simulink model "pmsm_sensorless_control"  (R2021a)
settings: Solver=VariableStepAuto  StartTime=0.0  StopTime=10.0  RelTol=1e-3
undefined symbols (not defined in the file): induction_motor, sin_cos_calculator
libraries: eeTransforms x2
settings Model: Creator=danesh  LastModifiedBy=danesh

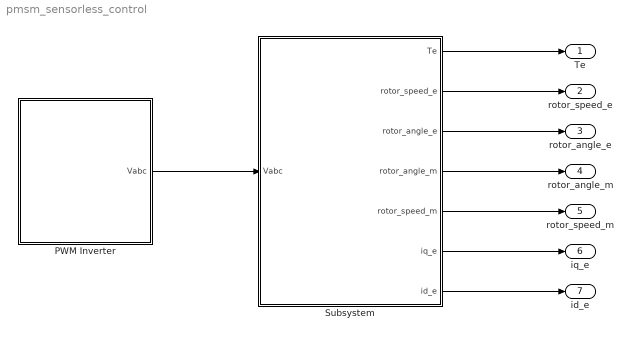
== system pmsm_sensorless_control ==
  PWM Inverter : Subsystem
  Subsystem : Subsystem
  Te : Outport  VectorParamsAs1DForOutWhenUnconnected=off
  rotor_speed_e : Outport  Port=2  VectorParamsAs1DForOutWhenUnconnected=off
  rotor_angle_e : Outport  Port=3  VectorParamsAs1DForOutWhenUnconnected=off
  rotor_angle_m : Outport  Port=4  VectorParamsAs1DForOutWhenUnconnected=off
  rotor_speed_m : Outport  Port=5  VectorParamsAs1DForOutWhenUnconnected=off
  iq_e : Outport  Port=6  VectorParamsAs1DForOutWhenUnconnected=off
  "id_e " : Outport  Port=7  VectorParamsAs1DForOutWhenUnconnected=off
  wires:
  Subsystem/6(iq_e) -> iq_e/1
  Subsystem/3(rotor_angle_e) -> rotor_angle_e/1
  Subsystem/5(rotor_speed_m) -> rotor_speed_m/1
  Subsystem/4(rotor_angle_m) -> rotor_angle_m/1
  Subsystem/2(rotor_speed_e) -> rotor_speed_e/1
  Subsystem/1(Te) -> Te/1
  PWM Inverter/1(Vabc) -> Subsystem/1(Vabc)
  Subsystem/7("id_e ") -> "id_e "/1

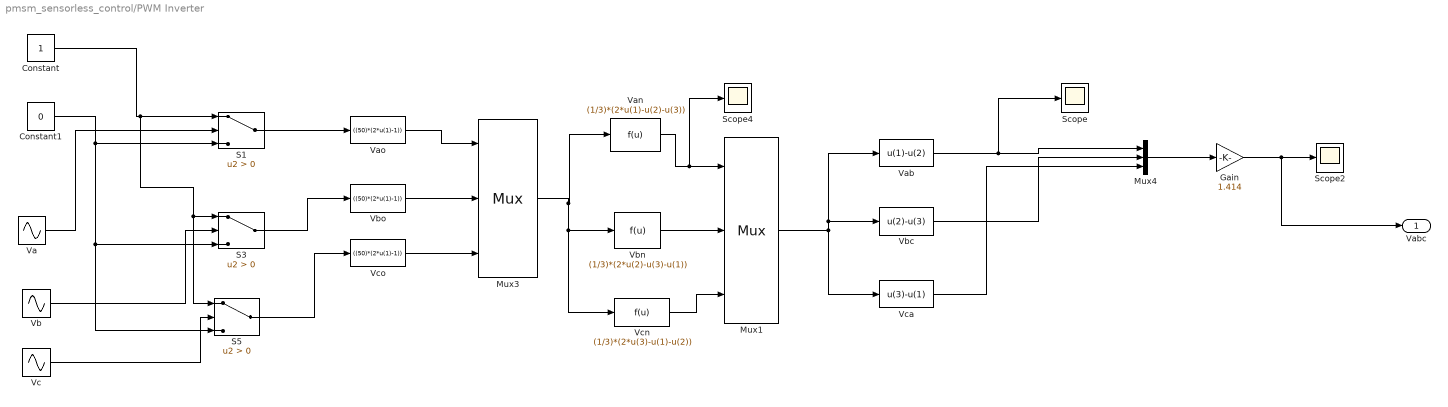
== system pmsm_sensorless_control/PWM Inverter ==
  Constant : Constant
  Constant1 : Constant  Value=0
  Gain : Gain  Gain=1.414
  Mux1 : Mux  Inputs=3
  Mux3 : Mux  Inputs=3
  Mux4 : Mux  Inputs=3
  S1 : Switch  Criteria=u2 > Threshold
  S3 : Switch  Criteria=u2 > Threshold
  S5 : Switch  Criteria=u2 > Threshold
  Scope : Scope
  Scope2 : Scope
  Scope4 : Scope
  Va : Sin  Frequency=2*pi*50  SampleTime=0
  Vab : Fcn  Expr=u(1)-u(2)
  Van : Fcn  Expr=(1/3)*(2*u(1)-u(2)-u(3))
  Vao : Fcn  Expr=((50)*(2*u(1)-1))
  Vb : Sin  Frequency=2*pi*50  Phase=-2.0904  SampleTime=0
  Vbc : Fcn  Expr=u(2)-u(3)
  Vbn : Fcn  Expr=(1/3)*(2*u(2)-u(3)-u(1))
  Vbo : Fcn  Expr=((50)*(2*u(1)-1))
  Vc : Sin  Frequency=2*pi*50  Phase=-4.188  SampleTime=0
  Vca : Fcn  Expr=u(3)-u(1)
  Vcn : Fcn  Expr=(1/3)*(2*u(3)-u(1)-u(2))
  Vco : Fcn  Expr=((50)*(2*u(1)-1))
  Vabc : Outport  VectorParamsAs1DForOutWhenUnconnected=off
  wires:
  S5/1 -> Vco/1
  S1/1 -> Vao/1
  Vca/1 -> Mux4/3
  Vc/1 -> S5/2
  Vb/1 -> S3/2
  Vab/1 -> Scope/1, Mux4/1
  Vbo/1 -> Mux3/2
  Van/1 -> Scope4/1, Mux1/1
  Mux4/1 -> Gain/1
  Gain/1 -> Vabc/1, Scope2/1
  Constant/1 -> S3/1, S5/1, S1/1
  Vco/1 -> Mux3/3
  Constant1/1 -> S1/3, S3/3, S5/3
  Mux3/1 -> Van/1, Vcn/1, Vbn/1
  S3/1 -> Vbo/1
  Mux1/1 -> Vbc/1, Vab/1, Vca/1
  Vao/1 -> Mux3/1
  Va/1 -> S1/2
  Vbn/1 -> Mux1/2
  Vcn/1 -> Mux1/3
  Vbc/1 -> Mux4/2

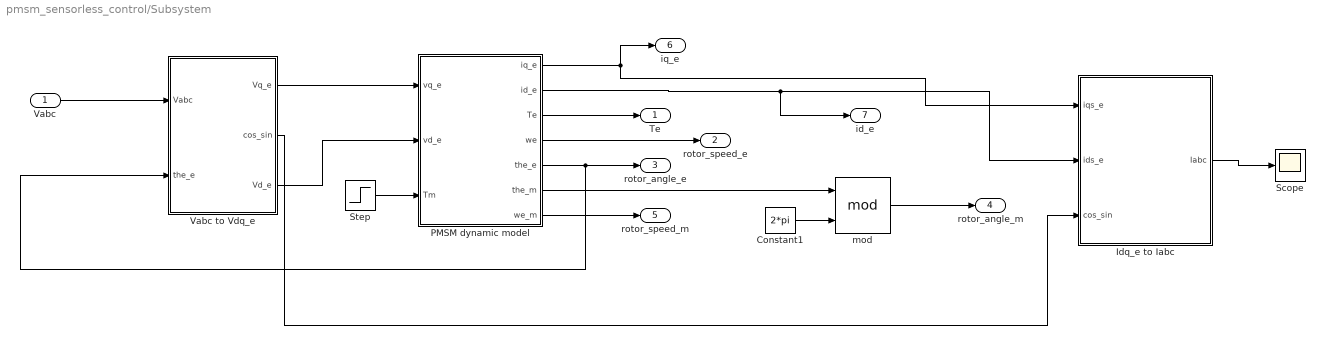
== system pmsm_sensorless_control/Subsystem ==
  Vabc : Inport
  Constant1 : Constant  Value=2*pi
  Idq_e to Iabc : Subsystem
  PMSM dynamic model : Subsystem
  Scope : Scope
  Step : Step  Time=3  SampleTime=0
  Vabc to Vdq_e : Subsystem
  mod : Math  Operator=mod  SignedPower=on  SaturateOnIntegerOverflow=on
  Te : Outport  VectorParamsAs1DForOutWhenUnconnected=off
  rotor_speed_e : Outport  Port=2  VectorParamsAs1DForOutWhenUnconnected=off
  rotor_angle_e : Outport  Port=3  VectorParamsAs1DForOutWhenUnconnected=off
  rotor_angle_m : Outport  Port=4  VectorParamsAs1DForOutWhenUnconnected=off
  rotor_speed_m : Outport  Port=5  VectorParamsAs1DForOutWhenUnconnected=off
  iq_e : Outport  Port=6  VectorParamsAs1DForOutWhenUnconnected=off
  "id_e " : Outport  Port=7  VectorParamsAs1DForOutWhenUnconnected=off
  wires:
  PMSM dynamic model/4(we) -> rotor_speed_e/1
  Idq_e to Iabc/1(Iabc) -> Scope/1
  PMSM dynamic model/2(id_e) -> "id_e "/1, Idq_e to Iabc/2(ids_e)
  mod/1 -> rotor_angle_m/1
  PMSM dynamic model/7(we_m) -> rotor_speed_m/1
  PMSM dynamic model/5(the_e) -> rotor_angle_e/1, Vabc to Vdq_e/2(the_e)
  PMSM dynamic model/6(the_m) -> mod/1
  Step/1 -> PMSM dynamic model/3(Tm)
  PMSM dynamic model/1(iq_e) -> iq_e/1, Idq_e to Iabc/1(iqs_e)
  PMSM dynamic model/3(Te) -> Te/1
  Constant1/1 -> mod/2
  Vabc to Vdq_e/1(Vq_e) -> PMSM dynamic model/1(vq_e)
  Vabc to Vdq_e/2(cos_sin) -> Idq_e to Iabc/3(cos_sin)
  Vabc to Vdq_e/3(Vd_e) -> PMSM dynamic model/2(vd_e)
  Vabc/1 -> Vabc to Vdq_e/1(Vabc)

== system pmsm_sensorless_control/Subsystem/Idq_e to Iabc ==
  iqs_e : Inport
  ids_e : Inport  Port=2
  cos_sin : Inport  Port=3
  Constant2 : Constant  Value=0
  Demux : Demux  Outputs=2
  Subsystem : Subsystem
  de-qe to ds-qs : Subsystem  AncestorBlock=induction_motor/de-qe to ds-qs
  Iabc : Outport  VectorParamsAs1DForOutWhenUnconnected=off
  wires:
  de-qe to ds-qs/1(qs_s) -> Subsystem/1(q_s)
  de-qe to ds-qs/2(ds_s) -> Subsystem/2(d_s)
  Constant2/1 -> Subsystem/4(thetha_degree)
  Subsystem/1(abc) -> Iabc/1
  iqs_e/1 -> de-qe to ds-qs/1(qs_e)
  ids_e/1 -> de-qe to ds-qs/2(ds_e)
  Demux/1 -> de-qe to ds-qs/3(cos Oe)
  Demux/2 -> de-qe to ds-qs/4(Sin Oe)
  cos_sin/1 -> Demux/1

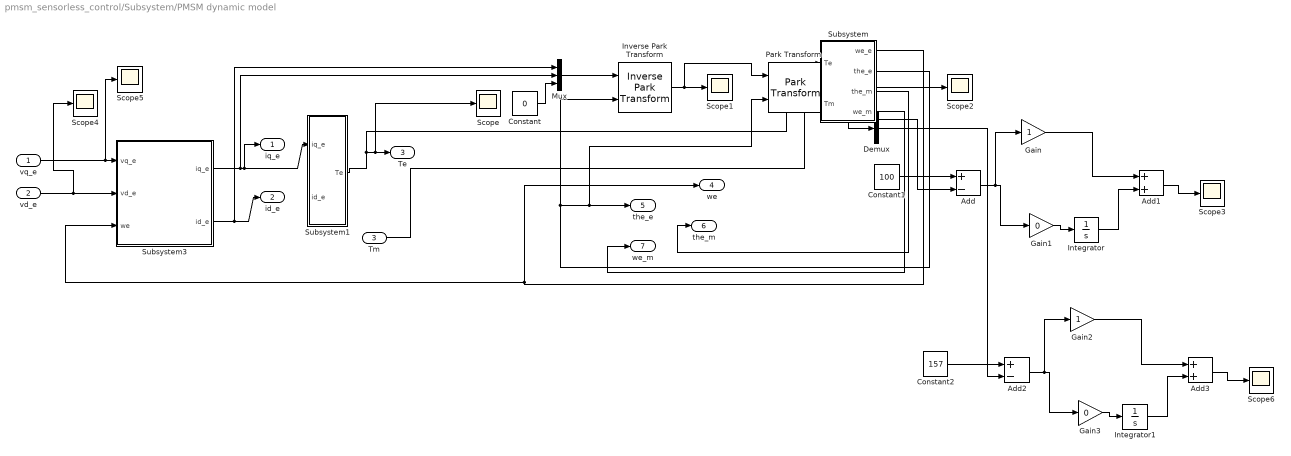
== system pmsm_sensorless_control/Subsystem/PMSM dynamic model ==
  vq_e : Inport
  vd_e : Inport  Port=2
  Tm : Inport  Port=3
  Add : Sum  Inputs=+-
  Add1 : Sum
  Add2 : Sum  Inputs=+-
  Add3 : Sum
  Constant : Constant  Value=0
  Constant1 : Constant  Value=100
  Constant2 : Constant  Value=157
  Demux : Demux  Outputs=3
  Gain : Gain
  Gain1 : Gain  Gain=0
  Gain2 : Gain
  Gain3 : Gain  Gain=0
  Integrator : Integrator
  Integrator1 : Integrator
  Inverse Park Transform : eeTransforms/Inverse Park Transform  AxisAlignment=Q-axis  PowerInvariant=off
  Mux : Mux  Inputs=3
  Park Transform : eeTransforms/Park Transform  AxisAlignment=Q-axis  PowerInvariant=off
  Scope{,1..6} (7 alike) : Scope
  Subsystem : Subsystem
  Subsystem1 : Subsystem
  Subsystem3 : Subsystem
  iq_e : Outport  VectorParamsAs1DForOutWhenUnconnected=off
  id_e : Outport  Port=2  VectorParamsAs1DForOutWhenUnconnected=off
  Te : Outport  Port=3  VectorParamsAs1DForOutWhenUnconnected=off
  we : Outport  Port=4  VectorParamsAs1DForOutWhenUnconnected=off
  the_e : Outport  Port=5  VectorParamsAs1DForOutWhenUnconnected=off
  the_m : Outport  Port=6  VectorParamsAs1DForOutWhenUnconnected=off
  we_m : Outport  Port=7  VectorParamsAs1DForOutWhenUnconnected=off
  wires:
  Subsystem1/1(Te) -> Subsystem/1(Te), Scope/1, Te/1
  Subsystem3/1(iq_e) -> Mux/2, Subsystem1/1(iq_e), iq_e/1
  Subsystem3/2(id_e) -> Mux/1, id_e/1
  Tm/1 -> Subsystem/2(Tm)
  vq_e/1 -> Scope5/1, Subsystem3/1(vq_e)
  vd_e/1 -> Scope4/1, Subsystem3/2(vd_e)
  Subsystem/2(the_e) -> Inverse Park Transform/2, Park Transform/2, the_e/1
  Subsystem/1(we_e) -> we/1, Subsystem3/3(we)
  Subsystem/3(the_m) -> the_m/1
  Subsystem/4(we_m) -> we_m/1
  Mux/1 -> Inverse Park Transform/1
  Constant/1 -> Mux/3
  Inverse Park Transform/1 -> Park Transform/1, Scope1/1
  Park Transform/1 -> Demux/1, Scope2/1
  Demux/1 -> Add/2
  Constant1/1 -> Add/1
  Add/1 -> Gain/1, Gain1/1
  Gain1/1 -> Integrator/1
  Gain/1 -> Add1/1
  Integrator/1 -> Add1/2
  Add1/1 -> Scope3/1
  Gain2/1 -> Add3/1
  Add3/1 -> Scope6/1
  Gain3/1 -> Integrator1/1
  Demux/2 -> Add2/2
  Constant2/1 -> Add2/1
  Add2/1 -> Gain2/1, Gain3/1
  Integrator1/1 -> Add3/2

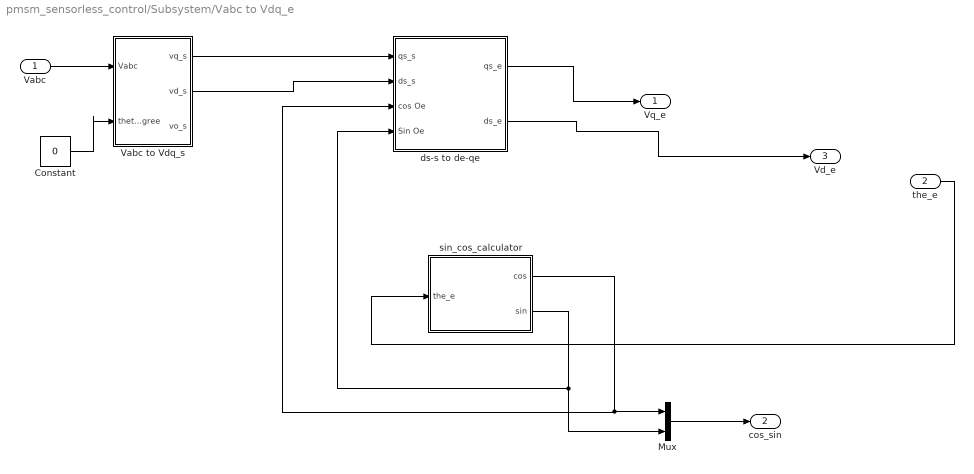
== system pmsm_sensorless_control/Subsystem/Vabc to Vdq_e ==
  Vabc : Inport
  the_e : Inport  Port=2
  Constant : Constant  Value=0
  Mux : Mux  Inputs=2
  Vabc to Vdq_s : Subsystem
  ds-s to de-qe : Subsystem  AncestorBlock=induction_motor/ds-s to de-qe
  sin_cos_calculator : Subsystem  AncestorBlock=induction_motor/sin_cos_calculator
  Vq_e : Outport  VectorParamsAs1DForOutWhenUnconnected=off
  cos_sin : Outport  Port=2  VectorParamsAs1DForOutWhenUnconnected=off
  Vd_e : Outport  Port=3  VectorParamsAs1DForOutWhenUnconnected=off
  wires:
  Mux/1 -> cos_sin/1
  sin_cos_calculator/1(cos) -> ds-s to de-qe/3(cos Oe), Mux/1
  Constant/1 -> Vabc to Vdq_s/2(thetha_degree)
  sin_cos_calculator/2(sin) -> Mux/2, ds-s to de-qe/4(Sin Oe)
  Vabc to Vdq_s/2(vd_s) -> ds-s to de-qe/2(ds_s)
  Vabc to Vdq_s/1(vq_s) -> ds-s to de-qe/1(qs_s)
  Vabc/1 -> Vabc to Vdq_s/1(Vabc)
  ds-s to de-qe/1(qs_e) -> Vq_e/1
  ds-s to de-qe/2(ds_e) -> Vd_e/1
  the_e/1 -> sin_cos_calculator/1(the_e)

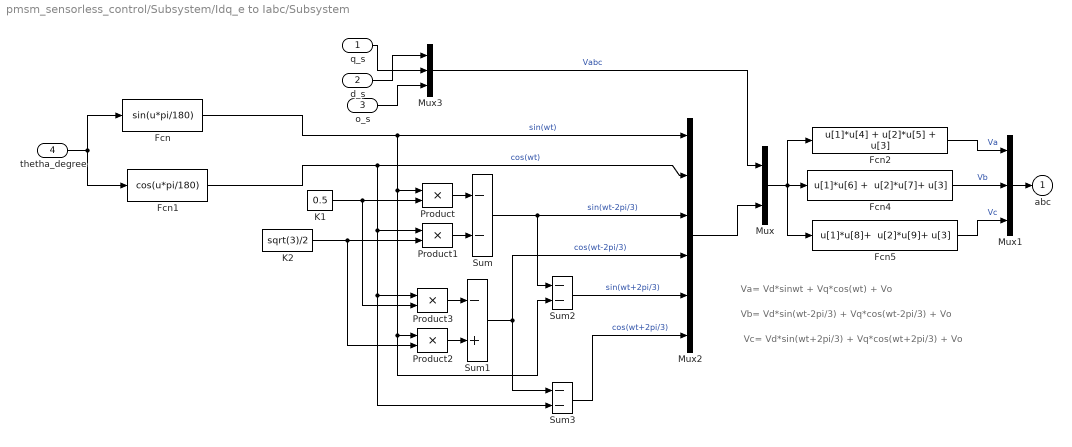
== system pmsm_sensorless_control/Subsystem/Idq_e to Iabc/Subsystem ==
  note: Va= Vd*sinwt + Vq*cos(wt) + Vo
  note: Vb= Vd*sin(wt-2pi/3) + Vq*cos(wt-2pi/3) + Vo
  note: Vc= Vd*sin(wt+2pi/3) + Vq*cos(wt+2pi/3) + Vo
  q_s : Inport
  d_s : Inport  Port=2
  o_s : Inport  Port=3
  thetha_degree : Inport  Port=4
  Fcn : Fcn  Expr=sin(u*pi/180)
  Fcn1 : Fcn  Expr=cos(u*pi/180)
  Fcn2 : Fcn  Expr="u[1]*u[4] +  u[2]*u[5] + u[3]"
  Fcn4 : Fcn  Expr="u[1]*u[6] +  u[2]*u[7]+ u[3]"
  Fcn5 : Fcn  Expr="u[1]*u[8]+  u[2]*u[9]+ u[3]"
  K1 : Constant  Value=0.5
  K2 : Constant  Value=sqrt(3)/2
  Mux : Mux  Inputs=2
  Mux1 : Mux  Inputs=3
  Mux2 : Mux  Inputs=6
  Mux3 : Mux  Inputs=3
  Product{,1..3} (4 alike) : Product  InputSameDT=on  SaturateOnIntegerOverflow=on  OutDataTypeStr=Inherit: Same as first input
  Sum : Sum  Inputs=--  InputSameDT=on  SaturateOnIntegerOverflow=on  OutDataTypeStr=Inherit: Same as first input
  Sum1 : Sum  Inputs=-+  InputSameDT=on  SaturateOnIntegerOverflow=on  OutDataTypeStr=Inherit: Same as first input
  Sum2 : Sum  Inputs=--  InputSameDT=on  SaturateOnIntegerOverflow=on  OutDataTypeStr=Inherit: Same as first input
  Sum3 : Sum  Inputs=--  InputSameDT=on  SaturateOnIntegerOverflow=on  OutDataTypeStr=Inherit: Same as first input
  abc : Outport  InitialOutput=0  VectorParamsAs1DForOutWhenUnconnected=off
  wires:
  o_s/1 -> Mux3/3
  q_s/1 -> Mux3/2
  d_s/1 -> Mux3/1
  Fcn5/1 -> Mux1/3  "Vc"
  Fcn2/1 -> Mux1/1  "Va"
  Mux1/1 -> abc/1
  Mux/1 -> Fcn4/1, Fcn2/1, Fcn5/1
  Sum1/1 -> Sum3/1, Mux2/4  "cos(wt-2pi/3)"
  Sum/1 -> Sum2/1, Mux2/3  "sin(wt-2pi/3)"
  K2/1 -> Product2/2, Product1/2
  K1/1 -> Product3/2, Product/2
  Sum2/1 -> Mux2/5  "sin(wt+2pi/3)"
  Sum3/1 -> Mux2/6  "cos(wt+2pi/3)"
  Product2/1 -> Sum1/2
  Product3/1 -> Sum1/1
  Product1/1 -> Sum/2
  Product/1 -> Sum/1
  Mux2/1 -> Mux/2
  Mux3/1 -> Mux/1  "Vabc"
  Fcn4/1 -> Mux1/2  "Vb"
  Fcn1/1 -> Mux2/2, Product1/1, Product3/1, Sum3/2  "cos(wt)"
  thetha_degree/1 -> Fcn/1, Fcn1/1
  Fcn/1 -> Mux2/1, Product/1, Sum2/2, Product2/1  "sin(wt)"

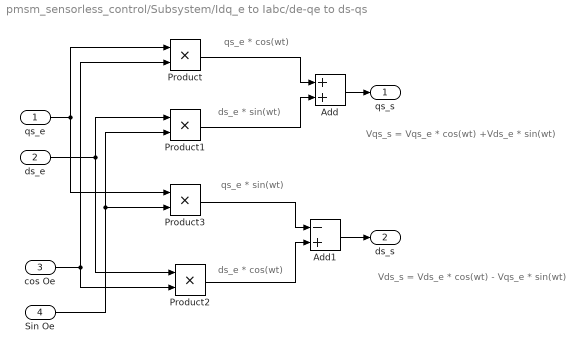
== system pmsm_sensorless_control/Subsystem/Idq_e to Iabc/de-qe to ds-qs ==
  note: Vds_s = Vds_e * cos(wt) - Vqs_e * sin(wt)
  note: Vqs_s = Vqs_e * cos(wt) +Vds_e * sin(wt)
  note: ds_e * cos(wt)
  note: qs_e * sin(wt)
  note: ds_e * sin(wt)
  note: qs_e * cos(wt)
  qs_e : Inport
  ds_e : Inport  Port=2
  cos Oe : Inport  Port=3
  Sin Oe : Inport  Port=4
  Add : Sum
  Add1 : Sum  Inputs=-+
  Product{,1..3} (4 alike) : Product  RndMeth=Zero
  qs_s : Outport  VectorParamsAs1DForOutWhenUnconnected=off
  ds_s : Outport  Port=2  VectorParamsAs1DForOutWhenUnconnected=off
  wires:
  Product/1 -> Add/1
  Product1/1 -> Add/2
  Product2/1 -> Add1/2
  Product3/1 -> Add1/1
  Add1/1 -> ds_s/1
  Add/1 -> qs_s/1
  Sin Oe/1 -> Product1/2, Product3/2
  ds_e/1 -> Product1/1, Product2/1
  cos Oe/1 -> Product/2, Product2/2
  qs_e/1 -> Product/1, Product3/1

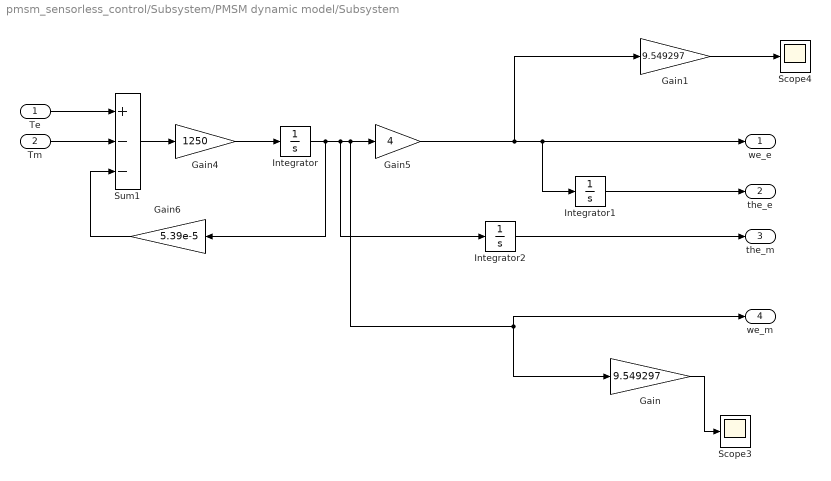
== system pmsm_sensorless_control/Subsystem/PMSM dynamic model/Subsystem ==
  Te : Inport
  Tm : Inport  Port=2
  Gain : Gain  Gain=9.549297
  Gain1 : Gain  Gain=9.549297
  Gain4 : Gain  Gain=1250  SaturateOnIntegerOverflow=on  OutDataTypeStr=Inherit: Same as input  ParamDataTypeStr=Inherit: Same as input
  Gain5 : Gain  Gain=4  SaturateOnIntegerOverflow=on  OutDataTypeStr=Inherit: Same as input  ParamDataTypeStr=Inherit: Same as input
  Gain6 : Gain  Gain=5.39e-5  SaturateOnIntegerOverflow=on  OutDataTypeStr=Inherit: Same as input  ParamDataTypeStr=Inherit: Same as input
  Integrator : Integrator
  Integrator1 : Integrator
  Integrator2 : Integrator
  Scope3 : Scope
  Scope4 : Scope
  Sum1 : Sum  Inputs=+--  InputSameDT=on  SaturateOnIntegerOverflow=on  OutDataTypeStr=Inherit: Same as first input
  we_e : Outport  VectorParamsAs1DForOutWhenUnconnected=off
  the_e : Outport  Port=2  VectorParamsAs1DForOutWhenUnconnected=off
  the_m : Outport  Port=3  VectorParamsAs1DForOutWhenUnconnected=off
  we_m : Outport  Port=4  VectorParamsAs1DForOutWhenUnconnected=off
  wires:
  Te/1 -> Sum1/1
  Tm/1 -> Sum1/2
  Sum1/1 -> Gain4/1
  Gain4/1 -> Integrator/1
  Gain6/1 -> Sum1/3
  Gain5/1 -> Gain1/1, Integrator1/1, we_e/1
  Integrator1/1 -> the_e/1
  Integrator2/1 -> the_m/1
  Integrator/1 -> Gain6/1, Integrator2/1, Gain5/1, Gain/1, we_m/1
  Gain/1 -> Scope3/1
  Gain1/1 -> Scope4/1

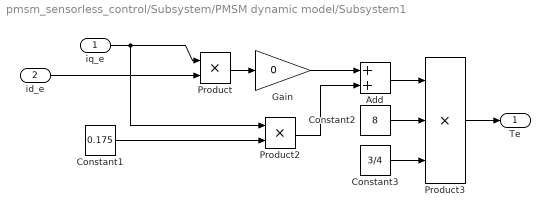
== system pmsm_sensorless_control/Subsystem/PMSM dynamic model/Subsystem1 ==
  iq_e : Inport
  id_e : Inport  Port=2
  Add : Sum
  Constant1 : Constant  Value=0.175
  Constant2 : Constant  Value=8
  Constant3 : Constant  Value=3/4
  Gain : Gain  Gain=0
  Product : Product  RndMeth=Zero
  Product2 : Product  RndMeth=Zero
  Product3 : Product  Inputs=3  RndMeth=Zero
  Te : Outport  VectorParamsAs1DForOutWhenUnconnected=off
  wires:
  iq_e/1 -> Product/1, Product2/1
  id_e/1 -> Product/2
  Product/1 -> Gain/1
  Constant1/1 -> Product2/2
  Gain/1 -> Add/1
  Product2/1 -> Add/2
  Add/1 -> Product3/1
  Constant2/1 -> Product3/2
  Constant3/1 -> Product3/3
  Product3/1 -> Te/1

== system pmsm_sensorless_control/Subsystem/PMSM dynamic model/Subsystem3 ==
  vq_e : Inport
  vd_e : Inport  Port=2
  we : Inport  Port=3
  Idq : Scope
  Mux : Mux  Inputs=2
  Subsystem1 : Subsystem
  Subsystem2 : Subsystem
  iq_e : Outport  VectorParamsAs1DForOutWhenUnconnected=off
  id_e : Outport  Port=2  VectorParamsAs1DForOutWhenUnconnected=off
  wires:
  vq_e/1 -> Subsystem1/3(vq)
  vd_e/1 -> Subsystem2/3(vd)
  we/1 -> Subsystem1/2(we), Subsystem2/2(we)
  Subsystem1/1(iq) -> Subsystem2/1(iq), Mux/1, iq_e/1
  Subsystem2/1(id) -> Subsystem1/1(id), Mux/2, id_e/1
  Mux/1 -> Idq/1

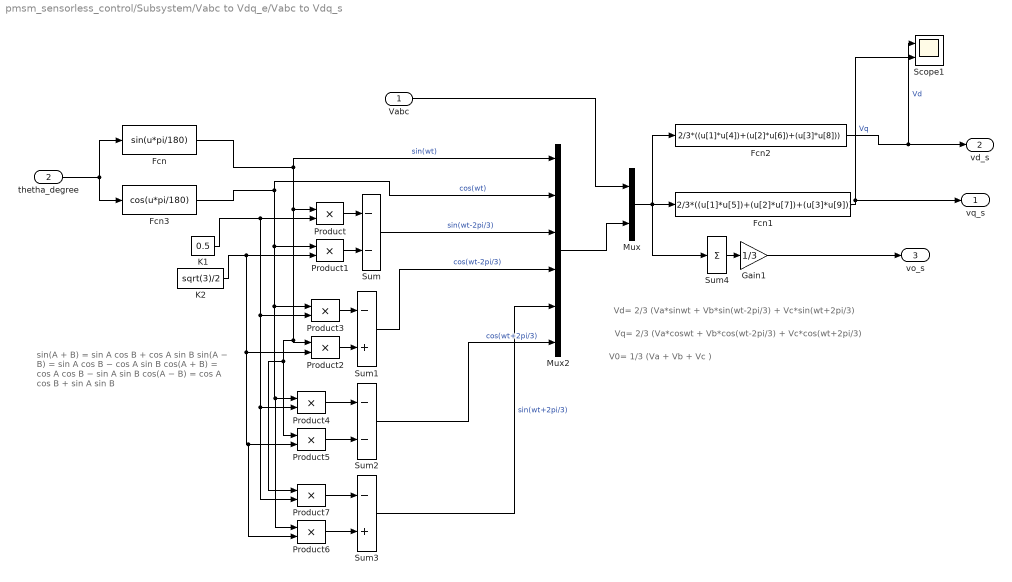
== system pmsm_sensorless_control/Subsystem/Vabc to Vdq_e/Vabc to Vdq_s ==
  note: Vd= 2/3 (Va*sinwt + Vb*sin(wt-2pi/3) + Vc*sin(wt+2pi/3)
  note: V0= 1/3 (Va + Vb + Vc )
  note: Vq= 2/3 (Va*coswt + Vb*cos(wt-2pi/3) + Vc*cos(wt+2pi/3)
  note: sin(A + B) = sin A cos B + cos A sin B
      | sin(A − B) = sin A cos B − cos A sin B
      | cos(A + B) = cos A cos B − sin A sin B
      | cos(A − B) = cos A cos B + sin A sin B
  Vabc : Inport
  thetha_degree : Inport  Port=2
  Fcn : Fcn  Expr=sin(u*pi/180)
  Fcn1 : Fcn  Expr=2/3*((u[1]*u[5])+(u[2]*u[7])+(u[3]*u[9]))
  Fcn2 : Fcn  Expr=2/3*((u[1]*u[4])+(u[2]*u[6])+(u[3]*u[8]))
  Fcn3 : Fcn  Expr=cos(u*pi/180)
  Gain1 : Gain  Gain=1/3  SaturateOnIntegerOverflow=on  OutDataTypeStr=Inherit: Same as input  ParamDataTypeStr=Inherit: Same as input
  K1 : Constant  Value=0.5
  K2 : Constant  Value=sqrt(3)/2
  Mux : Mux  Inputs=2
  Mux2 : Mux  Inputs=6
  Product{,1..7} (8 alike) : Product  InputSameDT=on  SaturateOnIntegerOverflow=on  OutDataTypeStr=Inherit: Same as first input
  Scope1 : Scope  NumInputPorts=2
  Sum : Sum  Inputs=--  InputSameDT=on  SaturateOnIntegerOverflow=on  OutDataTypeStr=Inherit: Same as first input
  Sum1 : Sum  Inputs=-+  InputSameDT=on  SaturateOnIntegerOverflow=on  OutDataTypeStr=Inherit: Same as first input
  Sum2 : Sum  Inputs=--  InputSameDT=on  SaturateOnIntegerOverflow=on  OutDataTypeStr=Inherit: Same as first input
  Sum3 : Sum  Inputs=-+  InputSameDT=on  SaturateOnIntegerOverflow=on  OutDataTypeStr=Inherit: Same as first input
  Sum4 : Sum  Inputs=1  InputSameDT=on  SaturateOnIntegerOverflow=on  OutDataTypeStr=Inherit: Same as first input
  vq_s : Outport  VectorParamsAs1DForOutWhenUnconnected=off
  vd_s : Outport  Port=2  VectorParamsAs1DForOutWhenUnconnected=off
  vo_s : Outport  Port=3  VectorParamsAs1DForOutWhenUnconnected=off
  wires:
  Product/1 -> Sum/1
  Fcn1/1 -> vq_s/1, Scope1/2  "Vq"
  K2/1 -> Product1/2, Product6/2, Product5/2, Product2/2
  Mux/1 -> Fcn2/1, Fcn1/1, Sum4/1
  Sum/1 -> Mux2/3  "sin(wt-2pi/3)"
  Fcn3/1 -> Product6/1, Product4/1, Product3/1, Product1/1, Mux2/2  "cos(wt)"
  K1/1 -> Product/2, Product7/2, Product4/2, Product3/2
  Product4/1 -> Sum2/1
  thetha_degree/1 -> Fcn3/1, Fcn/1
  Fcn/1 -> Product/1, Product7/1, Product5/1, Product2/1, Mux2/1  "sin(wt)"
  Product2/1 -> Sum1/2
  Product5/1 -> Sum2/2
  Sum3/1 -> Mux2/5  "sin(wt+2pi/3)"
  Product1/1 -> Sum/2
  Sum1/1 -> Mux2/4  "cos(wt-2pi/3)"
  Fcn2/1 -> vd_s/1, Scope1/1  "Vd"
  Gain1/1 -> vo_s/1
  Product6/1 -> Sum3/2
  Sum2/1 -> Mux2/6  "cos(wt+2pi/3)"
  Product7/1 -> Sum3/1
  Sum4/1 -> Gain1/1
  Mux2/1 -> Mux/2
  Product3/1 -> Sum1/1
  Vabc/1 -> Mux/1

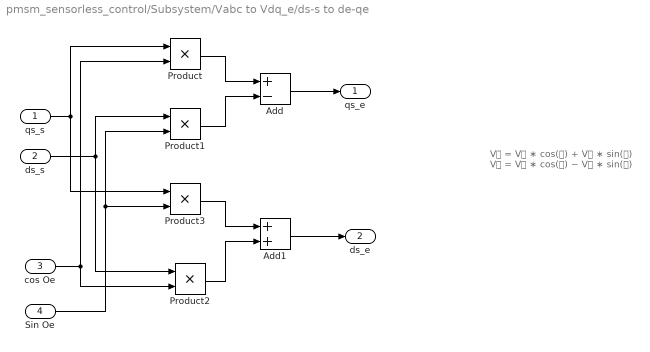
== system pmsm_sensorless_control/Subsystem/Vabc to Vdq_e/ds-s to de-qe ==
  note: V𝑑 = V𝛼 ∗ cos(𝜃) + V𝛽 ∗ sin(𝜃)
      |
      | V𝑞 = V𝛽 ∗ cos(𝜃) − V𝛼 ∗ sin(𝜃)
  qs_s : Inport
  ds_s : Inport  Port=2
  cos Oe : Inport  Port=3
  Sin Oe : Inport  Port=4
  Add : Sum  Inputs=+-
  Add1 : Sum
  Product{,1..3} (4 alike) : Product  RndMeth=Zero
  qs_e : Outport  VectorParamsAs1DForOutWhenUnconnected=off
  ds_e : Outport  Port=2  VectorParamsAs1DForOutWhenUnconnected=off
  wires:
  Product/1 -> Add/1
  Product1/1 -> Add/2
  Product2/1 -> Add1/2
  Product3/1 -> Add1/1
  Add1/1 -> ds_e/1
  Add/1 -> qs_e/1
  Sin Oe/1 -> Product1/2, Product3/2
  ds_s/1 -> Product1/1, Product2/1
  cos Oe/1 -> Product/2, Product2/2
  qs_s/1 -> Product/1, Product3/1

== system pmsm_sensorless_control/Subsystem/Vabc to Vdq_e/sin_cos_calculator ==
  the_e : Inport
  Fcn : Fcn  Expr=sin(u)
  Fcn1 : Fcn  Expr=cos(u)
  cos : Outport  VectorParamsAs1DForOutWhenUnconnected=off
  sin : Outport  Port=2  VectorParamsAs1DForOutWhenUnconnected=off
  wires:
  Fcn1/1 -> cos/1
  Fcn/1 -> sin/1
  the_e/1 -> Fcn/1, Fcn1/1

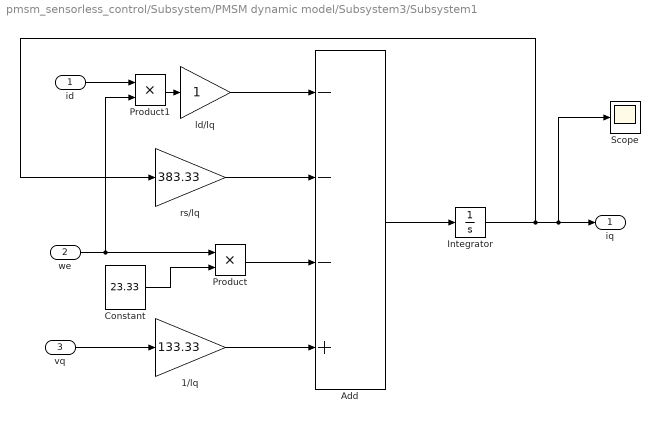
== system pmsm_sensorless_control/Subsystem/PMSM dynamic model/Subsystem3/Subsystem1 ==
  id : Inport
  we : Inport  Port=2
  vq : Inport  Port=3
  "1/lq " : Gain  Gain=133.33
  Add : Sum  Inputs=---+
  Constant : Constant  Value=23.33
  Integrator : Integrator
  Product : Product  RndMeth=Zero
  Product1 : Product  RndMeth=Zero
  Scope : Scope
  "ld/lq " : Gain
  rs/lq : Gain  Gain=383.33
  iq : Outport  VectorParamsAs1DForOutWhenUnconnected=off
  wires:
  vq/1 -> "1/lq "/1
  "ld/lq "/1 -> Add/1
  rs/lq/1 -> Add/2
  "1/lq "/1 -> Add/4
  Add/1 -> Integrator/1
  Integrator/1 -> rs/lq/1, Scope/1, iq/1
  Product/1 -> Add/3
  we/1 -> Product/1, Product1/2
  Constant/1 -> Product/2
  Product1/1 -> "ld/lq "/1
  id/1 -> Product1/1

== system pmsm_sensorless_control/Subsystem/PMSM dynamic model/Subsystem3/Subsystem2 ==
  iq : Inport
  we : Inport  Port=2
  vd : Inport  Port=3
  Add : Sum  Inputs=+-+
  Gain : Gain
  Gain1 : Gain  Gain=383.33
  Gain2 : Gain  Gain=133.33
  Integrator : Integrator
  Product : Product  RndMeth=Zero
  id : Outport  VectorParamsAs1DForOutWhenUnconnected=off
  wires:
  iq/1 -> Product/1
  we/1 -> Product/2
  Product/1 -> Gain/1
  Gain/1 -> Add/1
  Add/1 -> Integrator/1
  Gain1/1 -> Add/2
  vd/1 -> Gain2/1
  Gain2/1 -> Add/3
  Integrator/1 -> Gain1/1, id/1
